simulink model "openmodel"  (R2024b)
settings: Solver=ode4  StartTime=0.0  StopTime=20  FixedStep=0.001  RelTol=1e-3
undefined symbols (not defined in the file): A, Af, bt, Cd0, Cmq, CNa, Cnr, dmdt, fin_angles, fin_positions, gravity, L, me, mf, N, ni, r_cp, rho, Thrust
libraries: simulink x2, aerolibanim x1, shared6dof x1, matrix_library x1
settings Model: Creator=tanel  LastModifiedBy=tanel
settings DataIOCC: ReturnWorkspaceOutputs=off

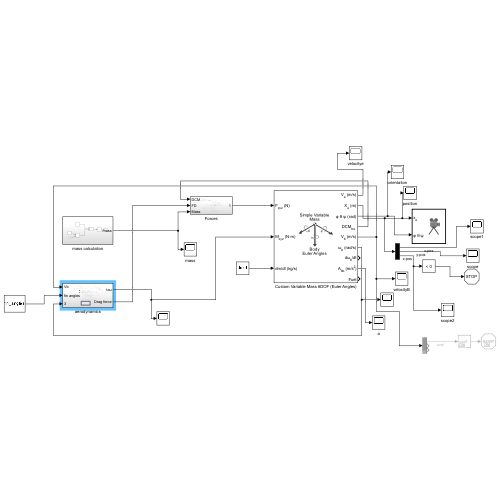
[thumbnail: Simulink's stored preview of the top-level diagram]
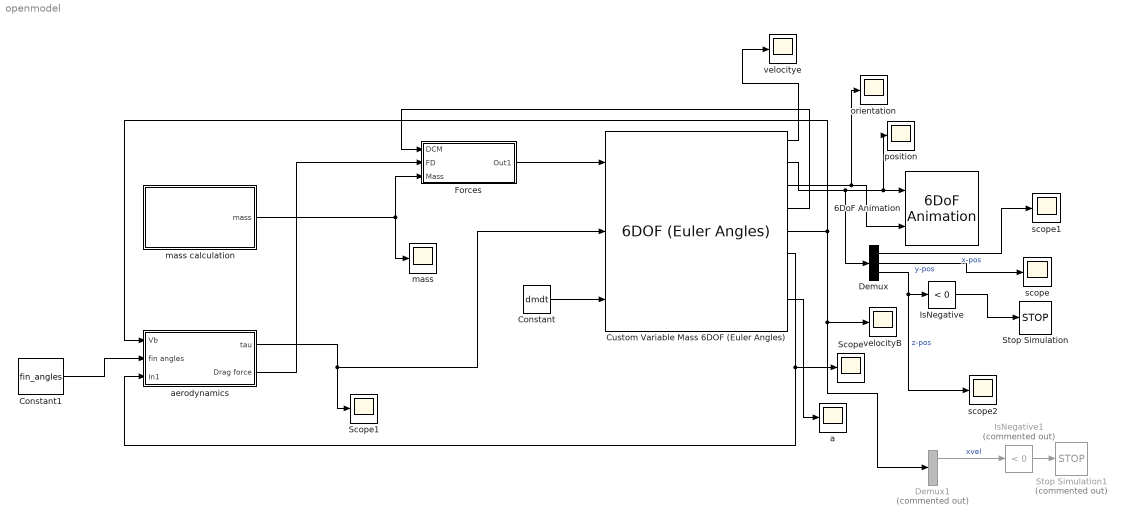
== system openmodel ==
  6DoF Animation : aerolibanim/6DoF Animation  u1=[0 40 -20 20 0 30]  u2=0.05  u3=1  u4=[400 0 -500]  u5=Fly alongside  u6=[0 10 0]  u7=10  u8=on
  Constant : Constant  Value=dmdt
  Constant1 : Constant  Value=fin_angles
  Custom Variable Mass 6DOF (Euler Angles) : shared6dof/6DOF (Euler Angles)  units=Metric (MKS)  mtype=Simple Variable  rep=Euler Angles  xme_0=[0 0 0]  Vm_0=[0.001 0 0]  eul_0=[0 -pi/2 0]  pm_0=[0 0 0]  mass_0=mf  mass_e=me  mass_f=mf  inertia=eye(3)  inertia_e=Ie  inertia_f=If  k_quat=1.0  vre_flag=off  abi_flag=off  aMode=0  xme_statename=''  Vm_statename=''  eul_statename=''  quat_statename=''  pm_statename=''  mass_statename=''
      settings: LibrarySourceBlock=aerolib6dof2/Custom Variable Mass 6DOF (Euler Angles)
  Demux : Demux  Outputs=3
  Demux1 : Demux  Commented=on  Outputs=3
  Forces : Subsystem
  IsNegative : simulink/Logic and Bit Operations/Compare To Zero  relop=<  OutDataTypeStr=boolean
      settings: LibrarySourceBlock=|
      | simulink/Quick Insert/Logic and Bit
      | Operations/IsNegative
  IsNegative1 : simulink/Logic and Bit Operations/Compare To Zero  Commented=on  relop=<  OutDataTypeStr=boolean
      settings: LibrarySourceBlock=|
      | simulink/Quick Insert/Logic and Bit
      | Operations/IsNegative
  Scope : Scope
  Scope1 : Scope
  Stop Simulation : Stop
  Stop Simulation1 : Stop  Commented=on
  a : Scope
  aerodynamics : Subsystem
  mass : Scope
  mass calculation : Subsystem
  orientation : Scope
  position : Scope
  scope : Scope
  scope1 : Scope
  scope2 : Scope
  velocityB : Scope
  velocitye : Scope
  wires:
  Constant/1 -> Custom Variable Mass 6DOF (Euler Angles)/3
  Custom Variable Mass 6DOF (Euler Angles)/4 -> Forces/1(DCM)
  Custom Variable Mass 6DOF (Euler Angles)/5 -> velocityB/1, Demux1/1, aerodynamics/1(Vb)
  Forces/1(Out1) -> Custom Variable Mass 6DOF (Euler Angles)/1
  aerodynamics/1(tau) -> Scope1/1, Custom Variable Mass 6DOF (Euler Angles)/2
  Custom Variable Mass 6DOF (Euler Angles)/3 -> orientation/1, 6DoF Animation/2
  Custom Variable Mass 6DOF (Euler Angles)/2 -> Demux/1, position/1, 6DoF Animation/1
  Demux/3 -> scope2/1, IsNegative/1  "z-pos"
  IsNegative/1 -> Stop Simulation/1
  Demux/2 -> scope/1  "y-pos"
  Demux/1 -> scope1/1  "x-pos"
  mass calculation/1(mass) -> mass/1, Forces/3(Mass)
  Custom Variable Mass 6DOF (Euler Angles)/1 -> velocitye/1
  Custom Variable Mass 6DOF (Euler Angles)/8 -> a/1
  Custom Variable Mass 6DOF (Euler Angles)/6 -> aerodynamics/3(In1), Scope/1
  Constant1/1 -> aerodynamics/2(fin angles)
  IsNegative1/1 -> Stop Simulation1/1
  Demux1/1 -> IsNegative1/1  "xvel"
  aerodynamics/2(Drag force) -> Forces/2(FD)

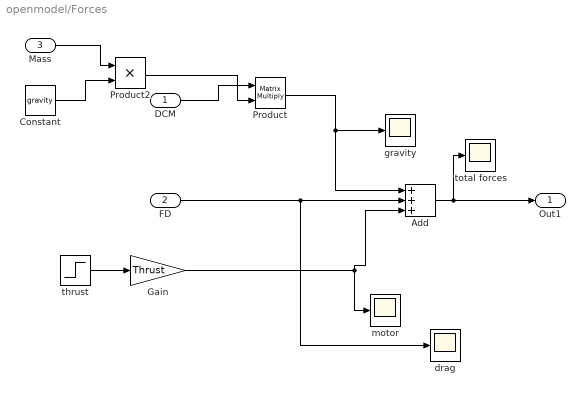
== system openmodel/Forces ==
  DCM : Inport
  FD : Inport  Port=2
  Mass : Inport  Port=3
  Add : Sum  Inputs=+|+|+
  Constant : Constant  Value=gravity  VectorParams1D=off
  Gain : Gain  Gain=Thrust
  Product : Product  Multiplication=Matrix(*)
  Product2 : Product
  drag : Scope
  gravity : Scope
  motor : Scope
  thrust : Step  Time=bt  Before=1  After=0  SampleTime=0  VectorParams1D=off
  total forces : Scope
  Out1 : Outport
  wires:
  Add/1 -> total forces/1, Out1/1
  Gain/1 -> Add/3, motor/1
  Constant/1 -> Product2/2
  Mass/1 -> Product2/1
  thrust/1 -> Gain/1
  Product/1 -> Add/1, gravity/1
  DCM/1 -> Product/1
  Product2/1 -> Product/2
  FD/1 -> drag/1, Add/2

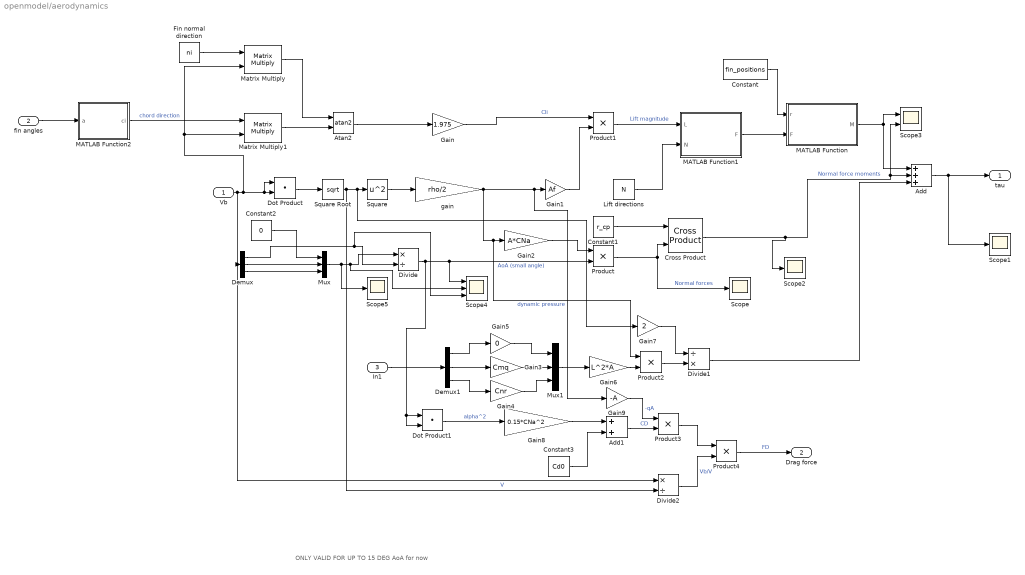
== system openmodel/aerodynamics ==
  note: ONLY VALID FOR UP TO 15 DEG AoA for now
  Vb : Inport
  fin angles : Inport  Port=2
  In1 : Inport  Port=3
  Add : Sum  Inputs=+++
  Add1 : Sum
  Atan2 : Trigonometry  Operator=atan2
  Constant : Constant  Value=fin_positions
  Constant1 : Constant  Value=r_cp
  Constant2 : Constant  Value=0
  Constant3 : Constant  Value=Cd0
  Cross Product : matrix_library/Cross Product
  Demux : Demux  Outputs=3
  Demux1 : Demux  Outputs=3
  Divide : Product  Inputs=*/
  Divide1 : Product  Inputs=/*
  Divide2 : Product  Inputs=*/
  Dot Product : DotProduct  OutDataTypeStr=Inherit: Inherit via internal rule
  Dot Product1 : DotProduct  OutDataTypeStr=Inherit: Inherit via internal rule
  Fin normal direction : Constant  Value=ni
  Gain : Gain  Gain=1.975
  Gain1 : Gain  Gain=Af
  Gain2 : Gain  Gain=A*CNa
  Gain3 : Gain  Gain=Cmq
  Gain4 : Gain  Gain=Cnr
  Gain5 : Gain  Gain=0
  Gain6 : Gain  Gain=L^2*A
  Gain7 : Gain  Gain=2
  Gain8 : Gain  Gain=0.15*CNa^2
  Gain9 : Gain  Gain=-A
  Lift directions : Constant  Value=N
  MATLAB Function : MATLAB Function  TreatAsAtomicUnit=on
  MATLAB Function1 : MATLAB Function  TreatAsAtomicUnit=on
  MATLAB Function2 : MATLAB Function  TreatAsAtomicUnit=on
  Matrix Multiply : Product  Multiplication=Matrix(*)
  Matrix Multiply1 : Product  Multiplication=Matrix(*)
  Mux : Mux  Inputs=3
  Mux1 : Mux  Inputs=3
  Product{,1..4} (5 alike) : Product
  Scope{,1..2,5} (4 alike) : Scope
  Scope3 : Scope  NumInputPorts=2
  Scope4 : Scope  NumInputPorts=3
  Square : Math  Operator=square
  Square Root : Sqrt
  gain : Gain  Gain=rho/2
  tau : Outport
  Drag force : Outport  Port=2
  wires:
  Square Root/1 -> Divide2/2, Gain7/1, Square/1  "V"
  Vb/1 -> Divide2/1, Demux/1, Dot Product/1, Dot Product/2, Matrix Multiply1/2, Matrix Multiply/2
  Constant/1 -> MATLAB Function/1(r)
  Gain/1 -> Product1/1  "Cli"
  gain/1 -> Product2/1, Gain2/1, Gain9/1, Gain1/1  "dynamic pressure"
  Product1/1 -> MATLAB Function1/1(L)  "Lift magnitude"
  Lift directions/1 -> MATLAB Function1/2(N)
  MATLAB Function1/1(F) -> MATLAB Function/2(F)
  Matrix Multiply/1 -> Atan2/1
  Matrix Multiply1/1 -> Atan2/2
  Atan2/1 -> Gain/1
  Fin normal direction/1 -> Matrix Multiply/1
  Dot Product/1 -> Square Root/1
  MATLAB Function2/1(ci) -> Matrix Multiply1/1  "chord direction"
  fin angles/1 -> MATLAB Function2/1(a)
  Square/1 -> gain/1
  Gain1/1 -> Product1/2
  Demux/2 -> Mux/2
  Demux/3 -> Mux/3
  Constant2/1 -> Mux/1
  Mux/1 -> Scope5/1, Scope4/2, Divide/1
  Demux/1 -> Scope4/3, Divide/2
  Divide/1 -> Dot Product1/1, Dot Product1/2, Scope4/1, Product/2  "AoA (small angle)"
  Gain2/1 -> Product/1
  Constant1/1 -> Cross Product/1
  Product/1 -> Scope/1, Cross Product/2  "Normal forces"
  Cross Product/1 -> Scope2/1, Scope3/2, Add/2  "Normal force moments"
  MATLAB Function/1(M) -> Add/1, Scope3/1
  Add/1 -> Scope1/1, tau/1
  In1/1 -> Demux1/1
  Demux1/2 -> Gain3/1
  Demux1/3 -> Gain4/1
  Demux1/1 -> Gain5/1
  Gain3/1 -> Mux1/2
  Gain4/1 -> Mux1/3
  Gain5/1 -> Mux1/1
  Mux1/1 -> Gain6/1
  Gain6/1 -> Product2/2
  Product2/1 -> Divide1/2
  Gain7/1 -> Divide1/1
  Divide1/1 -> Add/3
  Dot Product1/1 -> Gain8/1  "alpha^2"
  Constant3/1 -> Add1/2
  Gain8/1 -> Add1/1
  Add1/1 -> Product3/2  "CD"
  Gain9/1 -> Product3/1  "-qA"
  Divide2/1 -> Product4/2  "Vb/V"
  Product3/1 -> Product4/1
  Product4/1 -> Drag force/1  "FD"

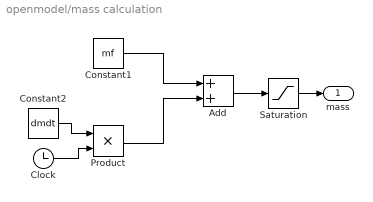
== system openmodel/mass calculation ==
  Add : Sum  OutMin=me
  Clock : Clock
  Constant1 : Constant  Value=mf
  Constant2 : Constant  Value=dmdt
  Product : Product
  Saturation : Saturate  UpperLimit=mf  LowerLimit=me
  mass : Outport
  wires:
  Add/1 -> Saturation/1
  Constant1/1 -> Add/1
  Product/1 -> Add/2
  Clock/1 -> Product/2
  Saturation/1 -> mass/1
  Constant2/1 -> Product/1

== matlab function openmodel/aerodynamics/MATLAB Function1 ==
  data: L input; F output; N input
function F = scaleForces(L,N)

F = L .* N;

end

== matlab function openmodel/aerodynamics/MATLAB Function ==
  data: r input; M output; F input
function M = computeTorque(r,F)

M = [0 0 0];

for i = 1:4
    M = M + cross(r(i,:), F(i,:));
end

end

== matlab function openmodel/aerodynamics/MATLAB Function2 ==
  data: a input; ci output
function ci = chordDirections(a)
    ci = [cos(a(1)) sin(a(1)) 0; cos(a(2)) 0 sin(a(2)); cos(a(3)) sin(a(3)) 0; cos(a(4)) 0 sin(a(4))];
end
